simulink model "MPC_UC_Exp_bj"  (R2016a)
settings: Solver=ode45  StartTime=0.0  StopTime=3830  RelTol=1e-3
StartFcn:
  | % clear all
libraries: mpclib x1, realtime_pacer_lib x1
settings Model: Creator=johnh  LastModifiedBy=tiago
settings DataIOCC: SaveFormat=StructureWithTime
settings OptimizationCC: BlockReduction=off  DefaultParameterBehavior=Inlined  BufferReuse=off
settings HardwareCC: ProdWordSize=32  ProdHWDeviceType=Specified
settings ConfigComp: CovModelRefEnable=Off

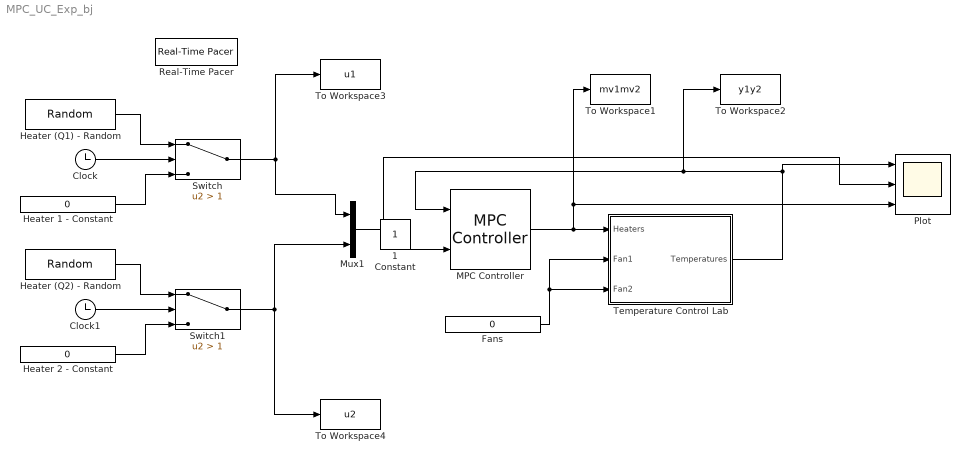
== system MPC_UC_Exp_bj ==
  Clock : Clock
  Clock1 : Clock
  Fans : Constant  Value=0
  Heater (Q1) - Random : RandomNumber  Mean=50  Variance=200  Seed=7  SampleTime=766
  Heater (Q2) - Random : RandomNumber  Mean=50  Variance=200  Seed=8  SampleTime=766
  Heater 1 - Constant : Constant  Value=0
  Heater 2 - Constant : Constant  Value=0
  MPC Controller : mpclib/MPC Controller  SCDEnableBlockLinearizationSpecification=on  mpcobj=MPC_UC_tclab_exp_bj  is_multiple=0  enable_value=0  return_u0=off  ref_from_ws=off  ref_signal_name=[]  ref_preview=off  md_from_ws=off  md_signal_name=[]  md_preview=off  from_project=off  project_file=MPCtask.mat  md_inport=off  mv_inport=off  cost_outport=off  return_sequence=off  return_qpstatus=off  return_state=off  state_inport=off  lims_inport=off  ywt_inport=off  is_designfromscratch=0  uwt_inport=off  duwt_inport=off  rhoeps_inport=off  uref_inport=off  n_ts=7  n_mv=2  n_md=0  n_ud=0  n_mo=2  n_uo=0  BlockDataType=double  SampleTimeInherited=off  switch_inport=off
  Mux1 : Mux  Inputs=2
  Plot : Scope  NumInputPorts=3
  Real-Time Pacer : realtime_pacer_lib/Real-Time Pacer  simTimePerRealTime=1
  Switch : Switch  Criteria=u2 > Threshold  Threshold=1
  Switch1 : Switch  Criteria=u2 > Threshold  Threshold=1
  Temperature Control Lab : Subsystem
      mask Display: image('tclab.png');
  To Workspace1 : ToWorkspace  VariableName=mv1mv2  SaveFormat=Timeseries  SampleTime=-1
  To Workspace2 : ToWorkspace  VariableName=y1y2  SaveFormat=Timeseries  SampleTime=-1
  To Workspace3 : ToWorkspace  VariableName=u1  SaveFormat=Timeseries  SampleTime=-1
  To Workspace4 : ToWorkspace  VariableName=u2  SaveFormat=Timeseries  SampleTime=-1
  1 : Constant  IOType=siggen
  Constant : Constant  IOType=siggen
  wires:
  MPC Controller/1 -> Plot/3, To Workspace1/1, Temperature Control Lab/1(Heaters)
  Fans/1 -> Temperature Control Lab/2(Fan1), Temperature Control Lab/3(Fan2)
  Heater (Q1) - Random/1 -> Switch/1
  Clock/1 -> Switch/2
  Heater 1 - Constant/1 -> Switch/3
  Heater (Q2) - Random/1 -> Switch1/1
  Clock1/1 -> Switch1/2
  Heater 2 - Constant/1 -> Switch1/3
  Switch/1 -> Mux1/1, To Workspace3/1
  Switch1/1 -> Mux1/2, To Workspace4/1
  Mux1/1 -> Plot/2, MPC Controller/2
  Temperature Control Lab/1(Temperatures) -> To Workspace2/1, MPC Controller/1, Plot/1

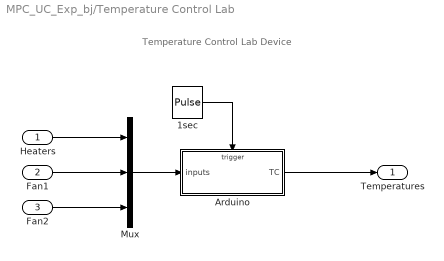
== system MPC_UC_Exp_bj/Temperature Control Lab ==
  note: Temperature Control Lab Device
  Heaters : Inport  PortDimensions=2
  Fan1 : Inport  Port=2  PortDimensions=1
  Fan2 : Inport  Port=3  PortDimensions=1
  1sec : DiscretePulseGenerator  PulseType=Time based  Period=0.5  PulseWidth=50
  Arduino : Subsystem  TreatAsAtomicUnit=on
  Mux : Mux  Inputs=3
  Temperatures : Outport
  wires:
  1sec/1 -> Arduino/Trigger
  Arduino/1(TC) -> Temperatures/1
  Mux/1 -> Arduino/1(inputs)
  Heaters/1 -> Mux/1
  Fan2/1 -> Mux/3
  Fan1/1 -> Mux/2

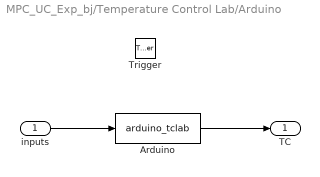
== system MPC_UC_Exp_bj/Temperature Control Lab/Arduino ==
  inputs : Inport  PortDimensions=4  LatchByDelayingOutsideSignal=on
  Trigger : TriggerPort  VariantControl=Variant
  Arduino : MATLABFcn  MATLABFcn=arduino_tclab
  TC : Outport  InitialOutput=[23 23]
  wires:
  inputs/1 -> Arduino/1
  Arduino/1 -> TC/1
